simulink model "ExampleModel"  (Simulink 7.8)
settings: Solver=FixedStepDiscrete  StartTime=0.0  StopTime=0.02  FixedStep=0.001  RelTol=1e-3
libraries: ExampleModel_lib x30, powerlib x5
settings Model: Creator=jde1  LastModifiedBy=jde1  BufferReuse=off
settings DataIOCC: LimitDataPoints=off  MaxDataPoints=1  SaveOutput=off  DSMLogging=off  SaveTime=off  StateSaveName=Display
settings OptimizationCC: OptimizeBlockIOStorage=off  BufferReuse=off  ExpressionFolding=off  LocalBlockOutputs=off

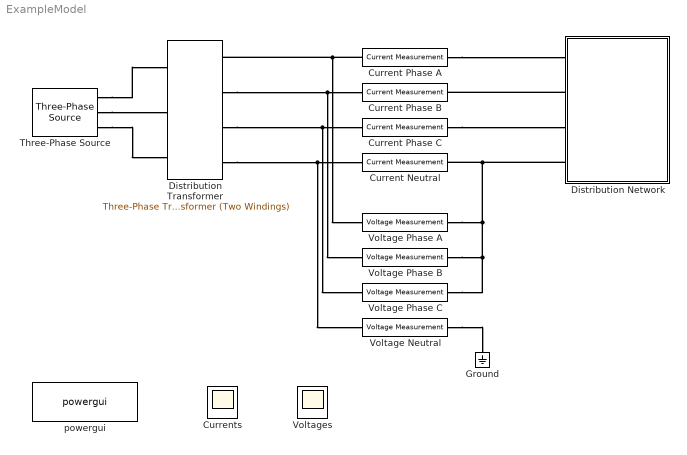
== system ExampleModel ==
  Current Neutral : ExampleModel_lib/Current Measurement  SystemSampleTime=-1
  Current Phase A : ExampleModel_lib/Current Measurement  SystemSampleTime=-1
  Current Phase B : ExampleModel_lib/Current Measurement  SystemSampleTime=-1
  Current Phase C : ExampleModel_lib/Current Measurement  SystemSampleTime=-1
  Currents : Scope
      settings: Floating=on  YMin=-150  YMax=150
  Distribution Transformer : powerlib/Elements/Three-Phase Transformer (Two Windings)  Winding1Connection=Yg  UNITS=SI  NominalPower=[ 300000 , 50 ]  Winding1=[22000 9.6316 0.30658]  Winding2Connection=Yn  Winding2=[440 0.0037656 0.00011986]  SetSaturation=off  Rm=1.21e+06  Lm=3851.5  Saturation=[0 0;0.030855 39.614;12.857 50.177]  Hysteresis=off  DataFile='hysteresis'  SetInitialFlux=off  InitialFluxes=[26.41 -26.41 23.108]  Measurements=None  MoreParameters=off  BreakLoop=off  DataType=on  TransfoNumber=1
  Distribution Network : Subsystem
  Ground : powerlib/Elements/Ground  LConnTagsString=a
  Three-Phase Source : powerlib/Electrical Sources/Three-Phase Source  Voltage=22000  PhaseAngle=0  Frequency=50  InternalConnection=Yg  SpecifyImpedance=off  Resistance=0.0001  Inductance=0.0001  ShortCircuitLevel=100e6  BaseVoltage=22000  XRratio=7  BusType=swing  Pref=0  Qref=0  Qmin=-inf  Qmax=inf
  Voltage Neutral : ExampleModel_lib/Voltage Measurement  SystemSampleTime=-1
  Voltage Phase A : ExampleModel_lib/Voltage Measurement  SystemSampleTime=-1
  Voltage Phase B : ExampleModel_lib/Voltage Measurement  SystemSampleTime=-1
  Voltage Phase C : ExampleModel_lib/Voltage Measurement  SystemSampleTime=-1
  Voltages : Scope
      settings: Floating=on  YMin=-350  YMax=350
  powergui : powerlib/powergui  Priority=1  SimulationMode=Discrete  SolverType=Backward Euler  SampleTime=0.001  frequency=60  SPID=off  DisableSnubberDevices=off  DisableRonSwitches=off  DisableVfSwitches=off  SwTol=0  Interpol=off  DisplayEquations=off  FunctionMessages=off  frequencyindice=50  Pbase=1e6  ErrMax=1e-4  Iterations=10  UnitsV=V  UnitsW=W  echomessages=on  HookPort=off  EnableUseOfTLC=off  x0status=steady  RestoreLinks=warning  ResistiveCurrentMeasurement=off  Ylog=off  Xlog=on  ShowGrid=off  save=off  variable=ZData  ZoomFFT=off  StartTime=0.0  cycles=1  DisplayStyle=1  FreqAxis=off  MaxFrequency=1000  frequencyindicesteady=1  RmsSteady=1  display=off  methode=off
  connections:
  Current Phase A/LConn1 -- Distribution Transformer/RConn1 -- Voltage Phase A/LConn1
  Distribution Transformer/RConn2 -- Current Phase B/LConn1 -- Voltage Phase B/LConn1
  Distribution Transformer/RConn3 -- Current Phase C/LConn1 -- Voltage Phase C/LConn1
  Distribution Transformer/RConn4 -- Current Neutral/RConn1 -- Voltage Neutral/LConn1
  Current Phase A/RConn1 -- Distribution Network/LConn1
  Distribution Network/LConn2 -- Current Phase B/RConn1
  Voltage Phase B/RConn1 -- Voltage Phase A/RConn1 -- Distribution Network/LConn4 -- Current Neutral/LConn1 -- Voltage Phase C/RConn1
  Current Phase C/RConn1 -- Distribution Network/LConn3
  Three-Phase Source/RConn1 -- Distribution Transformer/LConn1
  Three-Phase Source/RConn2 -- Distribution Transformer/LConn2
  Three-Phase Source/RConn3 -- Distribution Transformer/LConn3
  Voltage Neutral/RConn1 -- Ground/LConn1

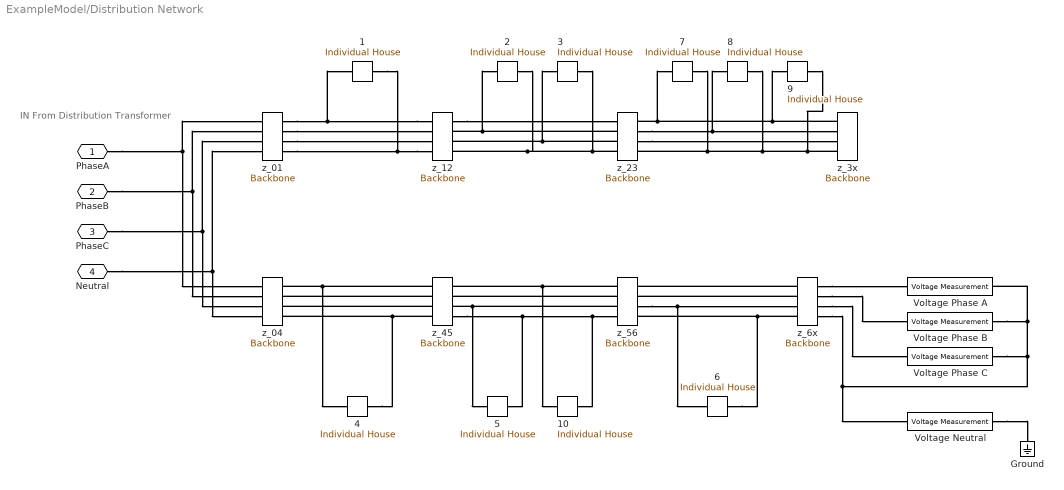
== system ExampleModel/Distribution Network ==
  note: IN From
      | Distribution
      | Transformer
  {1..10} (10 alike) : ExampleModel_lib/Individual House  length=0.025
  Ground : powerlib/Elements/Ground  LConnTagsString=a
  Voltage Neutral : ExampleModel_lib/Voltage Measurement  SystemSampleTime=-1
  Voltage Phase A : ExampleModel_lib/Voltage Measurement  SystemSampleTime=-1
  Voltage Phase B : ExampleModel_lib/Voltage Measurement  SystemSampleTime=-1
  Voltage Phase C : ExampleModel_lib/Voltage Measurement  SystemSampleTime=-1
  z_01 : ExampleModel_lib/Backbone  length=0.02
  z_04 : ExampleModel_lib/Backbone  length=0.02
  z_{12,23,45,56} (4 alike) : ExampleModel_lib/Backbone  length=0.02
  z_3x : ExampleModel_lib/Backbone  length=0.02
  z_6x : ExampleModel_lib/Backbone  length=0.02
  PhaseA : PMIOPort  Port=1  Side=Left
  PhaseB : PMIOPort  Port=2  Side=Left
  PhaseC : PMIOPort  Port=3  Side=Left
  Neutral : PMIOPort  Port=4  Side=Left
  connections:
  PhaseA/RConn1 -- z_01/LConn1 -- z_04/LConn1
  PhaseB/RConn1 -- z_01/LConn2 -- z_04/LConn2
  PhaseC/RConn1 -- z_01/LConn3 -- z_04/LConn3
  Neutral/RConn1 -- z_01/LConn4 -- z_04/LConn4
  z_12/LConn1 -- z_01/RConn1 -- 1/LConn1
  z_01/RConn2 -- z_12/LConn2
  z_01/RConn3 -- z_12/LConn3
  z_12/LConn4 -- z_01/RConn4 -- 1/RConn1
  z_12/RConn1 -- z_23/LConn1
  z_23/LConn2 -- z_12/RConn2 -- 2/LConn1
  z_23/LConn3 -- z_12/RConn3 -- 3/LConn1
  z_23/LConn4 -- z_12/RConn4 -- 2/RConn1 -- 3/RConn1
  z_45/LConn1 -- z_04/RConn1 -- 4/LConn1
  z_45/LConn2 -- z_04/RConn2
  z_45/LConn3 -- z_04/RConn3
  z_45/LConn4 -- z_04/RConn4 -- 4/RConn1
  z_56/LConn1 -- z_45/RConn1 -- 10/LConn1
  z_56/LConn2 -- z_45/RConn2
  z_56/LConn3 -- z_45/RConn3 -- 5/LConn1
  z_45/RConn4 -- 5/RConn1 -- z_56/LConn4 -- 10/RConn1
  z_23/RConn2 -- z_3x/LConn2 -- 8/LConn1
  z_3x/LConn4 -- z_23/RConn4 -- 7/RConn1 -- 8/RConn1 -- 9/RConn1
  z_23/RConn3 -- z_3x/LConn3
  z_3x/LConn1 -- z_23/RConn1 -- 7/LConn1 -- 9/LConn1
  z_56/RConn3 -- 6/LConn1 -- z_6x/LConn3
  z_56/RConn4 -- 6/RConn1 -- z_6x/LConn4
  z_6x/LConn2 -- z_56/RConn2
  z_6x/LConn1 -- z_56/RConn1
  Voltage Neutral/RConn1 -- Ground/LConn1
  z_6x/RConn1 -- Voltage Phase A/LConn1
  z_6x/RConn2 -- Voltage Phase B/LConn1
  z_6x/RConn3 -- Voltage Phase C/LConn1
  z_6x/RConn4 -- Voltage Neutral/LConn1 -- Voltage Phase C/RConn1 -- Voltage Phase B/RConn1 -- Voltage Phase A/RConn1
